simulink model "UAVVisualSLAMIn3DSimulation"  (R2024a)
settings: Solver=FixedStepAuto  StartTime=0.0  StopTime=pos(end,1)  RelTol=1e-3
StartFcn:
  | open_system([gcs, '/Video Viewer'])
values from neighbouring files (symbols this model uses):
  orientEuler = [0 0.05 0.1 0.15 0.2 0.25 0.3 0.35 0.4 0.45 0.5 0.55 ... (7988 elements, 1997x4)]    [uavStereoSLAMData.mat]
  pos = [0 0.05 0.1 0.15 0.2 0.25 0.3 0.35 0.4 0.45 0.5 0.55 ... (7988 elements, 1997x4)]    [uavStereoSLAMData.mat]
undefined symbols (not defined in the file or in its folder): baseline, gray
libraries: sim3dcameralib x2, sim3dlib x1, uavsim3dlib x1
settings Model: Creator=jianxins  LastModifiedBy=hrish
settings SolverCC: AlgebraicLoopSolver=TrustRegion
settings DataIOCC: SaveOutput=off  SignalLogging=off  DSMLogging=off
settings OptimizationCC: EnhancedBackFolding=on  PassReuseOutputArgsThreshold=0  MaxStackSize=64  OptimizeBlockOrder=speed  DifferentSizesBufferReuse=on  OptimizationCustomize=off
settings DebuggingCC: ParameterTunabilityLossMsg=error  UnconnectedInputMsg=warning  UnconnectedOutputMsg=warning  UnconnectedLineMsg=warning
settings HardwareCC: ProdBitPerPointer=32  ProdBitPerSizeT=32  ProdBitPerPtrDiffT=32  ProdLargestAtomicFloat=None  ProdIntDivRoundTo=Undefined  ProdEndianess=Unspecified  ProdWordSize=32  ProdHWDeviceType=Generic->Unspecified (assume 32-bit Generic)
settings ModelReferenceCC: EnableRefExpFcnMdlSchedulingChecks=on
settings SFSimCC: MATLABDynamicMemAlloc=off
settings RTWCC: Toolchain=Catkin  GPUComputeCapability=3.5  DLArmComputeVersion=19.05
settings CodeAppCC: ForceParamTrailComments=on  OperatorAnnotations=on
settings GRTTargetCC: TargetLangStandard=C89/C90 (ANSI)

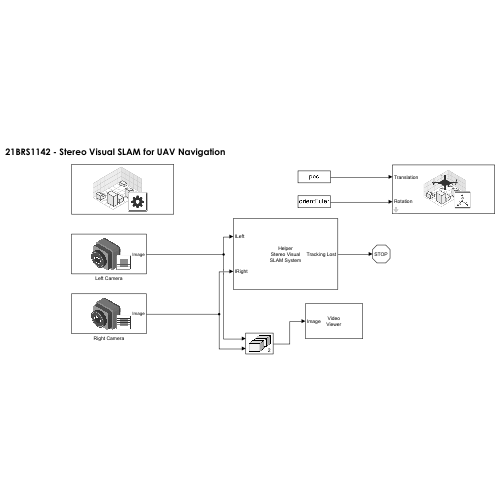
[thumbnail: Simulink's stored preview of the top-level diagram]
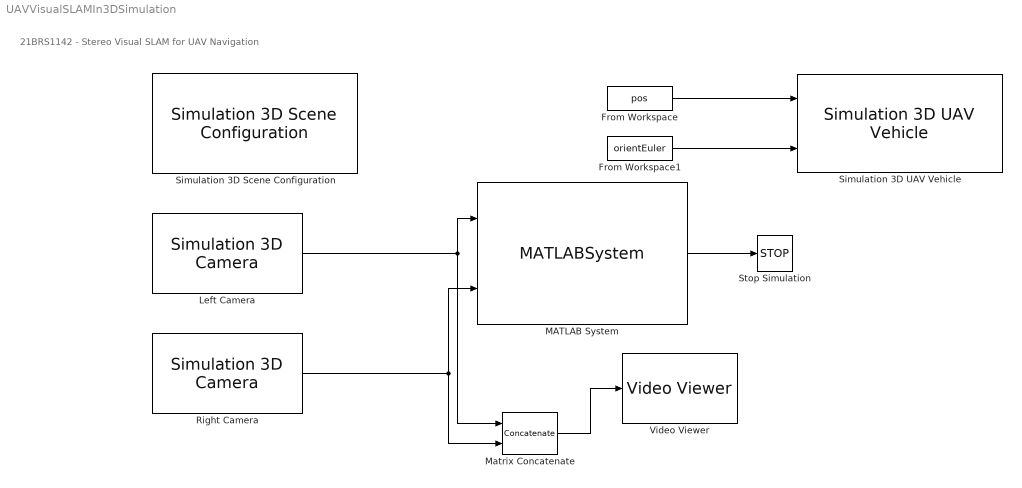
== system UAVVisualSLAMIn3DSimulation ==
  note: 21BRS1142 - Stereo Visual SLAM for UAV Navigation
  From Workspace : FromWorkspace  VariableName=pos
  From Workspace1 : FromWorkspace  VariableName=orientEuler
  Left Camera : sim3dcameralib/Simulation 3D Camera  Priority=1  sensorTag=Sim3dSensor1  sensorId=1  sensorName=Sim3dSensor1  vehTagList={'Scene Origin';'SimulinkVehicle1'}  vehTag=SimulinkVehicle1  mountLoc=Origin  offsetFlag=on  tmountOffset=[0, baseline/2, 0]  extTmount=off  rmountOffset=[0, 0, 0]  extRmount=off  FocalLength=focalLength  OpticalCenter=principalPoint  ImageSize=imageSize  RadialDistortion=[0, 0]  TangentialDistortion=[0, 0]  SensorSkew=0  DepthOutportEnabled=off  SemanticOutportEnabled=off  TransformOutportEnabled=off  SampleTime=-1  mountPoint=[0 -0.25 0]  mountOrientation=[0 0 0]  aMode=3  ID=1
      settings: LibrarySourceBlock=drivingsim3d/Simulation 3D Camera
  MATLAB System : MATLABSystem  System=HelperStereoVisualSLAMSystem  FocalLength=focalLength  PrincipalPoint=principalPoint  ImageSize=imageSize  Baseline=baseline  SimulateUsing=Interpreted execution
      mask Type: HelperStereoVisualSLAMSystem
      mask Display:
      | disp(['Helper' char(10) 'Stereo Visual' char(10) 'SLAM System']);
      | port_label('input',1,'ILeft');
      | port_label('input',2,'IRight');
      | port_label('output',1,'Tracking Lost');
  Matrix Concatenate : Concatenate  Mode=Multidimensional array  ConcatenateDimension=2
  Right Camera : sim3dcameralib/Simulation 3D Camera  Priority=1  sensorTag=Sim3dSensor2  sensorId=2  sensorName=Sim3dSensor2  vehTagList={'Scene Origin';'SimulinkVehicle1'}  vehTag=SimulinkVehicle1  mountLoc=Origin  offsetFlag=on  tmountOffset=[0, -baseline/2, 0]  extTmount=off  rmountOffset=[0, 0, 0]  extRmount=off  FocalLength=focalLength  OpticalCenter=principalPoint  ImageSize=imageSize  RadialDistortion=[0, 0]  TangentialDistortion=[0, 0]  SensorSkew=0  DepthOutportEnabled=off  SemanticOutportEnabled=off  TransformOutportEnabled=off  SampleTime=-1  mountPoint=[0 0.25 0]  mountOrientation=[0 0 0]  aMode=3  ID=2
      settings: LibrarySourceBlock=drivingsim3d/Simulation 3D Camera
  Simulation 3D Scene Configuration : sim3dlib/Simulation 3D Scene Configuration  Priority=0  ProjectFormat=Default Scenes  SceneDesc=US city block  ProjectName=C:\Program Files\MATLAB\R2024a\toolbox\shared\sim3d_projects\automotive_project_windows\UE\WindowsNoEditor\VehicleSimulation.exe  ScenePath=/Game/Maps/USCityBlock  EnableOpenDRIVE=off  vehTagList={'Custom';'Scene Origin';'SimulinkVehicle1'}  vehTag=SimulinkVehicle1  FreeCameraInitialTranslation=[0, 0, 0]  FreeCameraDefaultInitialTranslation=[-6, 0, 2]  FreeCameraInitialRotation=[0, 0, 0]  FreeCameraDefaultInitialRotation=[0, -15, 0]  OpVisEn=off  Ts=0.025  EnableWindow=off  EnableRemoteAccess=off  EnableWeather=on  SunAzimuth=90  SunAltitude=40.0  EnableGeospatialSun=off  Latitude=0  Longitude=0  Date=2023-01-01  Time=10:30:00  GeoTimeZone=-5.0  SunDaylightSaving=off  wind=1  clouds=20.0  EnableVolumetricClouds=off  CloudCoverage=0  CloudAltitude=6  fog=10.0  rain=10.0  RaindropsEffect=off  SnowDensity=0  EnableGeospatial=off  UseTrueOrigin=off  OriginHeight=200  OriginLatitude=40.744652  OriginLongitude=-73.988864  MapStyle=Aerial  AdditionalAssetIDs=[]  UseAdvancedSunSky=off  SolarTime=11  TimeZone=-5  Day=21  Month=9  Year=2022  UseDaylightSavingTime=on  DSTStartDay=10  DSTStartMonth=3  DSTEndDay=3  DSTEndMonth=11  DSTSwitchHour=2  sensorTag=MainCamera1  sensorId=1  sensorName=MainCamera1  mountLoc=Origin  offsetFlag=off  tmountOffset=[0, 0, 0]  rmountOffset=[0, 0, 0]  HorizontalResolution=1280  VerticalResolution=720  HorizontalFOV=60  mountPoint=[0 0 0]  mountOrientation=[0 0 0]  aMode=4  ID=1  GeoTrigger=Inactive
      settings: LibrarySourceBlock=uavsim3dlib/Simulation 3D Scene Configuration
  Simulation 3D UAV Vehicle : uavsim3dlib/Simulation 3D UAV Vehicle  Priority=-1  Mesh=Quadrotor  MeshPath=/MathWorksUAVContent/UAVs/HexaRotorUAV/HexaRotor.HexaRotor  Color=Black  ActorName=SimulinkVehicle1  UseGlobalFrame=off  InitialTranslation=pos(1,2:4)  InitialRotation=orientEuler(1,2:4)  InitialTranslationGlobal=[0 0 0]  InitialGeoOrigin=[0 0 0]  InitialRotationGlobal=[0 0 0]  SampleTime=-1  ActorType=SimulinkVehicle  ID=1  aMode=4  ActorTag=SimulinkVehicle1
  Stop Simulation : Stop
  Video Viewer : VideoViewer  colormapValue=gray(256)  FigPos=[33.8 483.6 974.4 344]
  wires:
  From Workspace/1 -> Simulation 3D UAV Vehicle/1
  From Workspace1/1 -> Simulation 3D UAV Vehicle/2
  Left Camera/1 -> Matrix Concatenate/1, MATLAB System/1
  Right Camera/1 -> Matrix Concatenate/2, MATLAB System/2
  Matrix Concatenate/1 -> Video Viewer/1
  MATLAB System/1 -> Stop Simulation/1
